simulink model "bai11"  (R2014a)
settings: Solver=ode45  StartTime=0.0  StopTime=10.0  RelTol=1e-3
libraries: powerlib x11
settings Model: Creator=503  LastModifiedBy=503

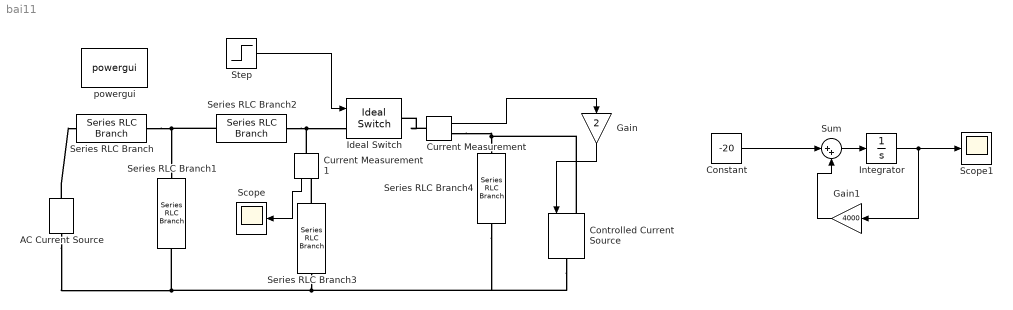
== system bai11 ==
  AC Current Source : powerlib/Electrical Sources/AC Current Source  Amplitude=10e-3  Phase=90  Frequency=0  SampleTime=0  Measurements=None
  Constant : Constant  Value=-20
  Controlled Current Source : powerlib/Electrical Sources/Controlled Current Source  Initialize=off  Source_Type=AC  Amplitude=0  Phase=0  Frequency=0  Measurements=None
  Current Measurement : powerlib/Measurements/Current Measurement  PhasorSimulation=off  OutputType=Complex  PSBequivalent=0
  Current Measurement1 : powerlib/Measurements/Current Measurement  PhasorSimulation=off  OutputType=Complex  PSBequivalent=0
  Gain : Gain  Gain=2
  Gain1 : Gain  Gain=4000
  Ideal Switch : powerlib/Power Electronics/Ideal Switch  Ron=1e-9  Lon=0  IC=0  Rs=inf  Cs=inf  Measurements=off
  Integrator : Integrator  InitialCondition=5e-3
  Scope : Scope
      settings: YMin=0.00499475  YMax=0.0049995
  Scope1 : Scope
      settings: YMin=-0.005  YMax=-0.005
  Series RLC Branch{,1..2,4} (4 alike) : powerlib/Elements/Series RLC Branch  LConnTagsString=__new0  RConnTagsString=__new0  BranchType=R  Resistance=2000  Inductance=1e-3  SetiL0=off  InitialCurrent=0  Capacitance=1e-6  Setx0=off  InitialVoltage=0  Measurements=None
  Series RLC Branch3 : powerlib/Elements/Series RLC Branch  LConnTagsString=__new0  RConnTagsString=__new0  BranchType=L  Resistance=2000  Inductance=2e-3  SetiL0=off  InitialCurrent=0  Capacitance=1e-6  Setx0=off  InitialVoltage=0  Measurements=None
  Step : Step  Time=0.1  SampleTime=0
  Sum : Sum  Inputs=|++
  powergui : powerlib/powergui  Priority=1  SimulationMode=Continuous  SolverType=Tustin  SampleTime=50e-6  frequency=60  SPID=off  DisableSnubberDevices=off  DisableRonSwitches=off  DisableVfSwitches=off  SwTol=0  Interpol=off  DisplayEquations=off  Ts=0  methode=off  frequencyindice=0  Pbase=100e6  ErrMax=1e-4  Iterations=50  UnitsV=kV  UnitsW=MW  FunctionMessages=off  echomessages=off  HookPort=off  EnableUseOfTLC=off  x0status=blocks  RestoreLinks=warning  ResistiveCurrentMeasurement=off  Frange=[0:2:500]  Ylog=off  Xlog=on  ShowGrid=off  save=off  variable=ZData  structure=0  ZoomFFT=off  StartTime=0.0  cycles=1  DisplayStyle=1  fundamental=60  FreqAxis=off  MaxFrequency=1000  frequencyindicesteady=1  RmsSteady=1  display=off
  wires:
  Current Measurement/1 -> Gain/1
  Gain/1 -> Controlled Current Source/1
  Current Measurement1/1 -> Scope/1
  Step/1 -> Ideal Switch/1
  Constant/1 -> Sum/1
  Gain1/1 -> Sum/2
  Sum/1 -> Integrator/1
  Integrator/1 -> Gain1/1, Scope1/1
  connections:
  Series RLC Branch/RConn1 -- Series RLC Branch2/RConn1 -- Series RLC Branch1/LConn1
  AC Current Source/LConn1 -- Series RLC Branch3/LConn1 -- Series RLC Branch4/RConn1 -- Controlled Current Source/RConn1 -- Series RLC Branch1/RConn1
  Series RLC Branch2/LConn1 -- Ideal Switch/LConn1 -- Current Measurement1/LConn1
  Current Measurement/RConn1 -- Controlled Current Source/LConn1 -- Series RLC Branch4/LConn1
  AC Current Source/RConn1 -- Series RLC Branch/LConn1
  Series RLC Branch3/RConn1 -- Current Measurement1/RConn1
  Current Measurement/LConn1 -- Ideal Switch/RConn1
